simulink model "flightControlSystem"  (R2024b)
settings: Solver=ode3  StartTime=0  StopTime=TFinal  FixedStep=Ts  RelTol=1e-3  EnableMultiTasking=on
undefined symbols (not defined in the file): codertarget, Controller, DiscIntNeverNeededParam, Discrete, Estimator, g, init, K, Sensors, Time, Ts, var_acc_angle_N, var_bias_gyr_N, var_gyro_p_N, Vehicle
libraries: simulink x51, slpidlib x16, sharedtransform x5, ctrlSharedLib x3, eeGeneralControl x1, parrotlib x1
(part 4 of 5)

== system flightControlSystem/Flight Control System/Subsystem/references/Attitude Controller ==
  note: Inner loop PID
      | controls angular velocity
  note: Outer Proportional loop
      | controls the pitch and roll angle
  note: ATTITUDE CONTROL
  refAttitude : Inport
  states_estim : Inport  Port=2
  Angle control loop : slpidlib/PID Controller  Controller=P  Form=Parallel  TimeDomain=Discrete-time  UseExternalTs=off  SampleTime=Ts  IntegratorMethod=Forward Euler  FilterMethod=Forward Euler  ControllerParametersSource=internal  P=2  I=1  UseKiTs=off  D=0  UseExternalDerivativeSource=off  N=100  UseFilter=on  TunerSelectOption=Transfer Function Based (PID Tuner App)  InitialConditionSource=internal  InitialConditionForIntegrator=0  InitialConditionForFilter=0  DifferentiatorICPrevScaledInput=0  ExternalReset=none  TrackingMode=off  Kt=1  LimitOutput=off  SatLimitsSource=internal  UpperSaturationLimit=inf  LowerSaturationLimit=-inf  LinearizeAsGain=on  AntiWindupMode=none  Kb=1  LimitIntegrator=off  UpperIntegratorSaturationLimit=inf  LowerIntegratorSaturationLimit=-inf  PGainOutDataTypeStr=single  PProdOutDataTypeStr=single  POutMin=[]  POutMax=[]  IOutMin=[]  IOutMax=[]  DOutMin=[]  DOutMax=[]  NOutMin=[]  NOutMax=[]  SumOutMin=[]  SumOutMax=[]  SaturationOutMin=[]  SaturationOutMax=[]  PParamMin=[]  PParamMax=[]  IParamMin=[]  IParamMax=[]  DParamMin=[]  DParamMax=[]  NParamMin=[]  NParamMax=[]  KbParamMin=[]  KbParamMax=[]  KtParamMin=[]  KtParamMax=[]  KbOutMin=[]  KbOutMax=[]  KtOutMin=[]  KtOutMax=[]  IntegratorOutMin=[]  IntegratorOutMax=[]  FilterOutMin=[]  FilterOutMax=[]  SumI1OutMin=[]  SumI1OutMax=[]  SumI2OutMin=[]  SumI2OutMax=[]  SumI3OutMin=[]  SumI3OutMax=[]  SumI4OutMin=[]  SumI4OutMax=[]  SumDOutMin=[]  SumDOutMax=[]  DifferentiatorOutMin=[]  DifferentiatorOutMax=[]  FilterDiffOutCoefMin=[]  FilterDiffOutCoefMax=[]  ReciprocalOutMin=[]  ReciprocalOutMax=[]  SumDenOutMin=[]  SumDenOutMax=[]  SumNumOutMin=[]  SumNumOutMax=[]  DivideOutMin=[]  DivideOutMax=[]  UdiffTsProdOutMin=[]  UdiffTsProdOutMax=[]  NTsProdOutMin=[]  NTsProdOutMax=[]  UintegralTsProdOutMin=[]  UintegralTsProdOutMax=[]  UngainTsProdOutMin=[]  UngainTsProdOutMax=[]  ClampingZeroOutDataTypeStr=Inherit: Inherit via back propagation  ClampingZeroOutMin=[]  ClampingZeroOutMax=[]  FilterDenConstantOutDataTypeStr=Inherit: Inherit via back propagation  FilterDenConstantOutMin=[]  FilterDenConstantOutMax=[]  PCopyOutDataTypeStr=Inherit: Inherit via back propagation  PCopyOutMin=[]  PCopyOutMax=[]  NCopyOutDataTypeStr=Inherit: Inherit via back propagation  NCopyOutMin=[]  NCopyOutMax=[]  IntegratorContinuousStateAttributes=''  IntegratorStateMustResolveToSignalObject=off  IntegratorRTWStateStorageClass=Auto  FilterContinuousStateAttributes=''  FilterStateMustResolveToSignalObject=off  FilterRTWStateStorageClass=Auto  ParallelPVariant=InternalParameters  IdealPVariant=Disabled  IVariant=Disabled  DVariant=Disabled  IntegratorVariant=Disabled  SatVariant=Disabled  AWVariant=Disabled  PCopyVariant=Disabled  TRVariant=Disabled  FdbkBlocksVariant=Forward  IdealPFdbkVariant=Disabled  SatFdbkVariant=Disabled  DerivativeFilterVariant=Disabled  NVariant=Disabled  NCopyVariant=Disabled_SignalSpec  FilterICVariant=Disabled  IntegratorICVariant=Disabled  ExternalResetVariant=Disabled  TRSumVariant=Passthrough  SumFdbkVariant=Disabled  SumVariant=Passthrough_P  TsampFilterVariant=InternalTs  TsampNgainVariant=Passthrough  TsampIntegralVariant=Disabled_SignalSpec  ExternalSaturationOutDataTypeStr=Inherit: Same as second input  DerivativeSourceVariant=Disabled  PreIntVariant=InternalPreInt
  Angular velocity control loop : slpidlib/PID Controller  Controller=PID  Form=Parallel  TimeDomain=Discrete-time  UseExternalTs=off  SampleTime=Ts  IntegratorMethod=Forward Euler  FilterMethod=Forward Euler  ControllerParametersSource=internal  P=0.003*[1 0.81]  I=2*0.003*[1 0.81]  UseKiTs=off  D=0.003/25*[1 0.81]  UseExternalDerivativeSource=off  N=70*[1 1]  UseFilter=on  TunerSelectOption=Transfer Function Based (PID Tuner App)  InitialConditionSource=internal  InitialConditionForIntegrator=0  InitialConditionForFilter=0  DifferentiatorICPrevScaledInput=0  ExternalReset=none  TrackingMode=off  Kt=1  LimitOutput=on  SatLimitsSource=internal  UpperSaturationLimit=0.02  LowerSaturationLimit=-0.02  LinearizeAsGain=on  AntiWindupMode=clamping  Kb=1  LimitIntegrator=off  UpperIntegratorSaturationLimit=inf  LowerIntegratorSaturationLimit=-inf  POutMin=[]  POutMax=[]  IOutMin=[]  IOutMax=[]  DOutMin=[]  DOutMax=[]  NOutMin=[]  NOutMax=[]  SumOutMin=[]  SumOutMax=[]  SaturationOutMin=[]  SaturationOutMax=[]  PParamMin=[]  PParamMax=[]  IParamMin=[]  IParamMax=[]  DParamMin=[]  DParamMax=[]  NParamMin=[]  NParamMax=[]  KbParamMin=[]  KbParamMax=[]  KtParamMin=[]  KtParamMax=[]  KbOutMin=[]  KbOutMax=[]  KtOutMin=[]  KtOutMax=[]  IntegratorOutMin=[]  IntegratorOutMax=[]  FilterOutMin=[]  FilterOutMax=[]  SumI1OutMin=[]  SumI1OutMax=[]  SumI2OutMin=[]  SumI2OutMax=[]  SumI3OutMin=[]  SumI3OutMax=[]  SumI4OutMin=[]  SumI4OutMax=[]  SumDOutMin=[]  SumDOutMax=[]  DifferentiatorOutMin=[]  DifferentiatorOutMax=[]  FilterDiffOutCoefMin=[]  FilterDiffOutCoefMax=[]  ReciprocalOutMin=[]  ReciprocalOutMax=[]  SumDenOutMin=[]  SumDenOutMax=[]  SumNumOutMin=[]  SumNumOutMax=[]  DivideOutMin=[]  DivideOutMax=[]  UdiffTsProdOutMin=[]  UdiffTsProdOutMax=[]  NTsProdOutMin=[]  NTsProdOutMax=[]  UintegralTsProdOutMin=[]  UintegralTsProdOutMax=[]  UngainTsProdOutMin=[]  UngainTsProdOutMax=[]  ClampingZeroOutDataTypeStr=Inherit: Inherit via back propagation  ClampingZeroOutMin=[]  ClampingZeroOutMax=[]  FilterDenConstantOutDataTypeStr=Inherit: Inherit via back propagation  FilterDenConstantOutMin=[]  FilterDenConstantOutMax=[]  PCopyOutDataTypeStr=Inherit: Inherit via back propagation  PCopyOutMin=[]  PCopyOutMax=[]  NCopyOutDataTypeStr=Inherit: Inherit via back propagation  NCopyOutMin=[]  NCopyOutMax=[]  IntegratorContinuousStateAttributes=''  IntegratorStateMustResolveToSignalObject=off  IntegratorRTWStateStorageClass=Auto  FilterContinuousStateAttributes=''  FilterStateMustResolveToSignalObject=off  FilterRTWStateStorageClass=Auto  ParallelPVariant=InternalParameters  IdealPVariant=Disabled  IVariant=InternalParameters  DVariant=InternalParameters  IntegratorVariant=Discrete  SatVariant=Enabled  AWVariant=DiscClampingParallel  PCopyVariant=Disabled  TRVariant=Disabled  FdbkBlocksVariant=Forward  IdealPFdbkVariant=Disabled  SatFdbkVariant=Disabled  DerivativeFilterVariant=ForwardEulerFilter  NVariant=InternalParameters  NCopyVariant=Disabled  FilterICVariant=InternalICsFilter  IntegratorICVariant=InternalICs  ExternalResetVariant=Disabled  TRSumVariant=Passthrough  SumFdbkVariant=Disabled  SumVariant=Sum_PID  TsampFilterVariant=InternalTs  TsampNgainVariant=Passthrough  TsampIntegralVariant=Disabled_SignalSpec  ExternalSaturationOutDataTypeStr=Inherit: Same as second input  DerivativeSourceVariant=ErrorSignal  PreIntVariant=InternalPreInt
  Bus Selector1 : BusSelector  OutputSignals=q,p
  Bus Selector3 : BusSelector  OutputSignals=pitch,roll
  Data Type Conversion : DataTypeConversion  SaturateOnIntegerOverflow=off  RndMeth=Floor
  Data Type Conversion1 : DataTypeConversion  SaturateOnIntegerOverflow=off  RndMeth=Floor
  Demux : Demux  Outputs=2
  Demux1 : Demux  Outputs=2
  Mux : Mux  Inputs=2
  Mux1 : Mux  Inputs=2
  Mux2 : Mux  Inputs=2
  Sum1 : Sum  Inputs=|+-
  Sum19 : Sum  Inputs=|+-
  tau_pitch : Outport  VectorParamsAs1DForOutWhenUnconnected=off
  tau_roll : Outport  Port=2  VectorParamsAs1DForOutWhenUnconnected=off
  angular velocity : Outport  Port=3
  wires:
  Sum1/1 -> Angular velocity control loop/1  "pitch/roll error"
  Angle control loop/1 -> Demux/1, Sum1/1
  Sum19/1 -> Angle control loop/1  "pitch/roll error"
  Angular velocity control loop/1 -> Data Type Conversion1/1
  Demux1/2 -> tau_roll/1  "roll acceleration"
  Demux1/1 -> tau_pitch/1  "pitch acceleration"
  Bus Selector3/2 -> Mux/2  "<roll>"
  refAttitude/1 -> Sum19/1
  Bus Selector3/1 -> Mux/1  "<pitch>"
  Bus Selector1/1 -> Mux2/1  "<q>"
  Bus Selector1/2 -> Mux2/2  "<p>"
  Demux/1 -> Mux1/2
  Demux/2 -> Mux1/1
  Mux1/1 -> Data Type Conversion/1
  states_estim/1 -> Bus Selector1/1, Bus Selector3/1
  Mux2/1 -> Sum1/2
  Mux/1 -> Sum19/2
  Data Type Conversion/1 -> angular velocity/1
  Data Type Conversion1/1 -> Demux1/1

== system flightControlSystem/Flight Control System/Subsystem/references/Position Controller ==
  note: Position controller requires good estimate of Yaw orientation to work properly.
      | Incase position control is not needed, the outer loop can be removed and velocity setpoint can be given directly
  note: Inner loop controls linear velocity error
  note: Outer loop controls the position error
  posXY : Inport
  states_estim : Inport  Port=2
  Bus Selector1 : BusSelector  OutputSignals=X,Y
  Bus Selector2 : BusSelector  OutputSignals=dx,dy
  Bus Selector3 : BusSelector  OutputSignals=yaw
  Data Type Conversion : DataTypeConversion  SaturateOnIntegerOverflow=off  RndMeth=Floor
  Data Type Conversion1 : DataTypeConversion  SaturateOnIntegerOverflow=off  RndMeth=Floor
  Gain : Gain  Gain=[-1, 1]
  LPF 8Hz Cutoff Filter to avoid oscillations induced by position controller : DiscreteTransferFcn  Numerator=[1, 1]  Denominator=[1+1/pi/Ts/8, 1-1/pi/Ts/8]
  Mux : Mux  Inputs=2
  Mux1 : Mux  Inputs=2
  Position controller : slpidlib/PID Controller  Controller=P  Form=Parallel  TimeDomain=Discrete-time  UseExternalTs=off  SampleTime=Ts  IntegratorMethod=Forward Euler  FilterMethod=Forward Euler  ControllerParametersSource=internal  P=0.7  I=0.1  UseKiTs=off  D=0  UseExternalDerivativeSource=off  N=100  UseFilter=on  TunerSelectOption=Transfer Function Based (PID Tuner App)  InitialConditionSource=internal  InitialConditionForIntegrator=0  InitialConditionForFilter=0  DifferentiatorICPrevScaledInput=0  ExternalReset=none  TrackingMode=off  Kt=1  LimitOutput=on  SatLimitsSource=internal  UpperSaturationLimit=0.5  LowerSaturationLimit=-0.5  LinearizeAsGain=on  AntiWindupMode=clamping  Kb=1  LimitIntegrator=off  UpperIntegratorSaturationLimit=inf  LowerIntegratorSaturationLimit=-inf  POutMin=[]  POutMax=[]  IOutMin=[]  IOutMax=[]  DOutMin=[]  DOutMax=[]  NOutMin=[]  NOutMax=[]  SumOutMin=[]  SumOutMax=[]  SaturationOutMin=[]  SaturationOutMax=[]  PParamMin=[]  PParamMax=[]  IParamMin=[]  IParamMax=[]  DParamMin=[]  DParamMax=[]  NParamMin=[]  NParamMax=[]  KbParamMin=[]  KbParamMax=[]  KtParamMin=[]  KtParamMax=[]  KbOutMin=[]  KbOutMax=[]  KtOutMin=[]  KtOutMax=[]  IntegratorOutMin=[]  IntegratorOutMax=[]  FilterOutMin=[]  FilterOutMax=[]  SumI1OutMin=[]  SumI1OutMax=[]  SumI2OutMin=[]  SumI2OutMax=[]  SumI3OutMin=[]  SumI3OutMax=[]  SumI4OutMin=[]  SumI4OutMax=[]  SumDOutMin=[]  SumDOutMax=[]  DifferentiatorOutMin=[]  DifferentiatorOutMax=[]  FilterDiffOutCoefMin=[]  FilterDiffOutCoefMax=[]  ReciprocalOutMin=[]  ReciprocalOutMax=[]  SumDenOutMin=[]  SumDenOutMax=[]  SumNumOutMin=[]  SumNumOutMax=[]  DivideOutMin=[]  DivideOutMax=[]  UdiffTsProdOutMin=[]  UdiffTsProdOutMax=[]  NTsProdOutMin=[]  NTsProdOutMax=[]  UintegralTsProdOutMin=[]  UintegralTsProdOutMax=[]  UngainTsProdOutMin=[]  UngainTsProdOutMax=[]  ClampingZeroOutDataTypeStr=Inherit: Inherit via back propagation  ClampingZeroOutMin=[]  ClampingZeroOutMax=[]  FilterDenConstantOutDataTypeStr=Inherit: Inherit via back propagation  FilterDenConstantOutMin=[]  FilterDenConstantOutMax=[]  PCopyOutDataTypeStr=Inherit: Inherit via back propagation  PCopyOutMin=[]  PCopyOutMax=[]  NCopyOutDataTypeStr=Inherit: Inherit via back propagation  NCopyOutMin=[]  NCopyOutMax=[]  IntegratorContinuousStateAttributes=''  IntegratorStateMustResolveToSignalObject=off  IntegratorRTWStateStorageClass=Auto  FilterContinuousStateAttributes=''  FilterStateMustResolveToSignalObject=off  FilterRTWStateStorageClass=Auto  ParallelPVariant=InternalParameters  IdealPVariant=Disabled  IVariant=Disabled  DVariant=Disabled  IntegratorVariant=Disabled  SatVariant=Enabled  AWVariant=Disabled  PCopyVariant=Disabled  TRVariant=Disabled  FdbkBlocksVariant=Forward  IdealPFdbkVariant=Disabled  SatFdbkVariant=Disabled  DerivativeFilterVariant=Disabled  NVariant=Disabled  NCopyVariant=Disabled_SignalSpec  FilterICVariant=Disabled  IntegratorICVariant=Disabled  ExternalResetVariant=Disabled  TRSumVariant=Passthrough  SumFdbkVariant=Disabled  SumVariant=Passthrough_P  TsampFilterVariant=InternalTs  TsampNgainVariant=Passthrough  TsampIntegralVariant=Disabled_SignalSpec  ExternalSaturationOutDataTypeStr=Inherit: Same as second input  DerivativeSourceVariant=Disabled  PreIntVariant=InternalPreInt
  Position error transformation (Earth to Body frame) : MATLAB Function  TreatAsAtomicUnit=on
  Sum1 : Sum  Inputs=|+-
  Sum19 : Sum  Inputs=|+-
  Velocity controller : slpidlib/PID Controller  Controller=PI  Form=Parallel  TimeDomain=Discrete-time  UseExternalTs=off  SampleTime=Ts  IntegratorMethod=Forward Euler  FilterMethod=Forward Euler  ControllerParametersSource=internal  P=0.2  I=0.1  UseKiTs=off  D=0  UseExternalDerivativeSource=off  N=100  UseFilter=on  TunerSelectOption=Transfer Function Based (PID Tuner App)  InitialConditionSource=internal  InitialConditionForIntegrator=0  InitialConditionForFilter=0  DifferentiatorICPrevScaledInput=0  ExternalReset=none  TrackingMode=off  Kt=1  LimitOutput=on  SatLimitsSource=internal  UpperSaturationLimit=20*pi/180  LowerSaturationLimit=-20*pi/180  LinearizeAsGain=on  AntiWindupMode=clamping  Kb=1  LimitIntegrator=off  UpperIntegratorSaturationLimit=inf  LowerIntegratorSaturationLimit=-inf  POutMin=[]  POutMax=[]  IOutMin=[]  IOutMax=[]  DOutMin=[]  DOutMax=[]  NOutMin=[]  NOutMax=[]  SumOutMin=[]  SumOutMax=[]  SaturationOutMin=[]  SaturationOutMax=[]  PParamMin=[]  PParamMax=[]  IParamMin=[]  IParamMax=[]  DParamMin=[]  DParamMax=[]  NParamMin=[]  NParamMax=[]  KbParamMin=[]  KbParamMax=[]  KtParamMin=[]  KtParamMax=[]  KbOutMin=[]  KbOutMax=[]  KtOutMin=[]  KtOutMax=[]  IntegratorOutMin=[]  IntegratorOutMax=[]  FilterOutMin=[]  FilterOutMax=[]  SumI1OutMin=[]  SumI1OutMax=[]  SumI2OutMin=[]  SumI2OutMax=[]  SumI3OutMin=[]  SumI3OutMax=[]  SumI4OutMin=[]  SumI4OutMax=[]  SumDOutMin=[]  SumDOutMax=[]  DifferentiatorOutMin=[]  DifferentiatorOutMax=[]  FilterDiffOutCoefMin=[]  FilterDiffOutCoefMax=[]  ReciprocalOutMin=[]  ReciprocalOutMax=[]  SumDenOutMin=[]  SumDenOutMax=[]  SumNumOutMin=[]  SumNumOutMax=[]  DivideOutMin=[]  DivideOutMax=[]  UdiffTsProdOutMin=[]  UdiffTsProdOutMax=[]  NTsProdOutMin=[]  NTsProdOutMax=[]  UintegralTsProdOutMin=[]  UintegralTsProdOutMax=[]  UngainTsProdOutMin=[]  UngainTsProdOutMax=[]  ClampingZeroOutDataTypeStr=Inherit: Inherit via back propagation  ClampingZeroOutMin=[]  ClampingZeroOutMax=[]  FilterDenConstantOutDataTypeStr=Inherit: Inherit via back propagation  FilterDenConstantOutMin=[]  FilterDenConstantOutMax=[]  PCopyOutDataTypeStr=Inherit: Inherit via back propagation  PCopyOutMin=[]  PCopyOutMax=[]  NCopyOutDataTypeStr=Inherit: Inherit via back propagation  NCopyOutMin=[]  NCopyOutMax=[]  IntegratorContinuousStateAttributes=''  IntegratorStateMustResolveToSignalObject=off  IntegratorRTWStateStorageClass=Auto  FilterContinuousStateAttributes=''  FilterStateMustResolveToSignalObject=off  FilterRTWStateStorageClass=Auto  ParallelPVariant=InternalParameters  IdealPVariant=Disabled  IVariant=InternalParameters  DVariant=Disabled  IntegratorVariant=Discrete  SatVariant=Enabled  AWVariant=DiscClampingParallel  PCopyVariant=Disabled  TRVariant=Disabled  FdbkBlocksVariant=Forward  IdealPFdbkVariant=Disabled  SatFdbkVariant=Disabled  DerivativeFilterVariant=Disabled  NVariant=Disabled  NCopyVariant=Disabled_SignalSpec  FilterICVariant=Disabled  IntegratorICVariant=InternalICs  ExternalResetVariant=Disabled  TRSumVariant=Passthrough  SumFdbkVariant=Disabled  SumVariant=Sum_PI  TsampFilterVariant=InternalTs  TsampNgainVariant=Passthrough  TsampIntegralVariant=Disabled_SignalSpec  ExternalSaturationOutDataTypeStr=Inherit: Same as second input  DerivativeSourceVariant=Disabled  PreIntVariant=InternalPreInt
  Velocity controller1 : slpidlib/PID Controller  Controller=PI  Form=Parallel  TimeDomain=Discrete-time  UseExternalTs=off  SampleTime=Ts  IntegratorMethod=Forward Euler  FilterMethod=Forward Euler  ControllerParametersSource=internal  P=0.7  I=0  UseKiTs=off  D=0  UseExternalDerivativeSource=off  N=100  UseFilter=on  TunerSelectOption=Transfer Function Based (PID Tuner App)  InitialConditionSource=internal  InitialConditionForIntegrator=0  InitialConditionForFilter=0  DifferentiatorICPrevScaledInput=0  ExternalReset=none  TrackingMode=off  Kt=1  LimitOutput=on  SatLimitsSource=internal  UpperSaturationLimit=20*pi/180  LowerSaturationLimit=-20*pi/180  LinearizeAsGain=on  AntiWindupMode=clamping  Kb=1  LimitIntegrator=off  UpperIntegratorSaturationLimit=inf  LowerIntegratorSaturationLimit=-inf  POutMin=[]  POutMax=[]  IOutMin=[]  IOutMax=[]  DOutMin=[]  DOutMax=[]  NOutMin=[]  NOutMax=[]  SumOutMin=[]  SumOutMax=[]  SaturationOutMin=[]  SaturationOutMax=[]  PParamMin=[]  PParamMax=[]  IParamMin=[]  IParamMax=[]  DParamMin=[]  DParamMax=[]  NParamMin=[]  NParamMax=[]  KbParamMin=[]  KbParamMax=[]  KtParamMin=[]  KtParamMax=[]  KbOutMin=[]  KbOutMax=[]  KtOutMin=[]  KtOutMax=[]  IntegratorOutMin=[]  IntegratorOutMax=[]  FilterOutMin=[]  FilterOutMax=[]  SumI1OutMin=[]  SumI1OutMax=[]  SumI2OutMin=[]  SumI2OutMax=[]  SumI3OutMin=[]  SumI3OutMax=[]  SumI4OutMin=[]  SumI4OutMax=[]  SumDOutMin=[]  SumDOutMax=[]  DifferentiatorOutMin=[]  DifferentiatorOutMax=[]  FilterDiffOutCoefMin=[]  FilterDiffOutCoefMax=[]  ReciprocalOutMin=[]  ReciprocalOutMax=[]  SumDenOutMin=[]  SumDenOutMax=[]  SumNumOutMin=[]  SumNumOutMax=[]  DivideOutMin=[]  DivideOutMax=[]  UdiffTsProdOutMin=[]  UdiffTsProdOutMax=[]  NTsProdOutMin=[]  NTsProdOutMax=[]  UintegralTsProdOutMin=[]  UintegralTsProdOutMax=[]  UngainTsProdOutMin=[]  UngainTsProdOutMax=[]  ClampingZeroOutDataTypeStr=Inherit: Inherit via back propagation  ClampingZeroOutMin=[]  ClampingZeroOutMax=[]  FilterDenConstantOutDataTypeStr=Inherit: Inherit via back propagation  FilterDenConstantOutMin=[]  FilterDenConstantOutMax=[]  PCopyOutDataTypeStr=Inherit: Inherit via back propagation  PCopyOutMin=[]  PCopyOutMax=[]  NCopyOutDataTypeStr=Inherit: Inherit via back propagation  NCopyOutMin=[]  NCopyOutMax=[]  IntegratorContinuousStateAttributes=''  IntegratorStateMustResolveToSignalObject=off  IntegratorRTWStateStorageClass=Auto  FilterContinuousStateAttributes=''  FilterStateMustResolveToSignalObject=off  FilterRTWStateStorageClass=Auto  ParallelPVariant=InternalParameters  IdealPVariant=Disabled  IVariant=InternalParameters  DVariant=Disabled  IntegratorVariant=Discrete  SatVariant=Enabled  AWVariant=DiscClampingParallel  PCopyVariant=Disabled  TRVariant=Disabled  FdbkBlocksVariant=Forward  IdealPFdbkVariant=Disabled  SatFdbkVariant=Disabled  DerivativeFilterVariant=Disabled  NVariant=Disabled  NCopyVariant=Disabled_SignalSpec  FilterICVariant=Disabled  IntegratorICVariant=InternalICs  ExternalResetVariant=Disabled  TRSumVariant=Passthrough  SumFdbkVariant=Disabled  SumVariant=Sum_PI  TsampFilterVariant=InternalTs  TsampNgainVariant=Passthrough  TsampIntegralVariant=Disabled_SignalSpec  ExternalSaturationOutDataTypeStr=Inherit: Same as second input  DerivativeSourceVariant=Disabled  PreIntVariant=InternalPreInt
  pitch_roll_cmd : Outport  VectorParamsAs1DForOutWhenUnconnected=off
  velocity_ref : Outport  Port=2
  acceleration_ref : Outport  Port=3
  wires:
  Bus Selector2/1 -> Mux1/1  "<dx>"
  states_estim/1 -> Bus Selector2/1, Bus Selector1/1, Bus Selector3/1
  Bus Selector1/1 -> Mux/1  "<X>"
  Bus Selector1/2 -> Mux/2  "<Y>"
  Bus Selector2/2 -> Mux1/2  "<dy>"
  Mux1/1 -> Sum19/2
  Sum19/1 -> Data Type Conversion1/1, Velocity controller/1
  Velocity controller/1 -> LPF 8Hz Cutoff Filter to avoid oscillations induced by position controller/1
  Gain/1 -> pitch_roll_cmd/1  "Pitch,Roll setpoint"
  LPF 8Hz Cutoff Filter to avoid oscillations induced by position controller/1 -> Gain/1
  Position controller/1 -> Data Type Conversion/1, Sum19/1  "Velocity  setpoint"
  Mux/1 -> Sum1/2
  Sum1/1 -> Position error transformation (Earth to Body frame)/2(xy_err_earth)
  Position error transformation (Earth to Body frame)/1(xy_err_body) -> Position controller/1
  posXY/1 -> Sum1/1  "Position setpoint"
  Bus Selector3/1 -> Position error transformation (Earth to Body frame)/1(yaw)  "<yaw>"
  Velocity controller1/1 -> acceleration_ref/1
  Data Type Conversion/1 -> velocity_ref/1
  Data Type Conversion1/1 -> Velocity controller1/1

== system flightControlSystem/Flight Control System/Controller1/Quaternion-based SMC attitude Controller/Angular velocity handling/Angular velocity ==
  note: Outer Proportional loop
      | controls the pitch and roll angle
  refAttitude1 : Inport
  states_estim1 : Inport  Port=2
  Angle control loop : slpidlib/PID Controller  Controller=P  Form=Parallel  TimeDomain=Discrete-time  UseExternalTs=off  SampleTime=Ts  IntegratorMethod=Forward Euler  FilterMethod=Forward Euler  ControllerParametersSource=internal  P=4  I=0  UseKiTs=off  D=0  UseExternalDerivativeSource=off  N=100  UseFilter=on  TunerSelectOption=Transfer Function Based (PID Tuner App)  InitialConditionSource=internal  InitialConditionForIntegrator=0  InitialConditionForFilter=0  DifferentiatorICPrevScaledInput=0  ExternalReset=none  TrackingMode=off  Kt=1  LimitOutput=off  SatLimitsSource=internal  UpperSaturationLimit=inf  LowerSaturationLimit=-inf  LinearizeAsGain=on  AntiWindupMode=none  Kb=1  LimitIntegrator=off  UpperIntegratorSaturationLimit=inf  LowerIntegratorSaturationLimit=-inf  POutMin=[]  POutMax=[]  IOutMin=[]  IOutMax=[]  DOutMin=[]  DOutMax=[]  NOutMin=[]  NOutMax=[]  SumOutMin=[]  SumOutMax=[]  SaturationOutMin=[]  SaturationOutMax=[]  PParamMin=[]  PParamMax=[]  IParamMin=[]  IParamMax=[]  DParamMin=[]  DParamMax=[]  NParamMin=[]  NParamMax=[]  KbParamMin=[]  KbParamMax=[]  KtParamMin=[]  KtParamMax=[]  KbOutMin=[]  KbOutMax=[]  KtOutMin=[]  KtOutMax=[]  IntegratorOutMin=[]  IntegratorOutMax=[]  FilterOutMin=[]  FilterOutMax=[]  SumI1OutMin=[]  SumI1OutMax=[]  SumI2OutMin=[]  SumI2OutMax=[]  SumI3OutMin=[]  SumI3OutMax=[]  SumI4OutMin=[]  SumI4OutMax=[]  SumDOutMin=[]  SumDOutMax=[]  DifferentiatorOutMin=[]  DifferentiatorOutMax=[]  FilterDiffOutCoefMin=[]  FilterDiffOutCoefMax=[]  ReciprocalOutMin=[]  ReciprocalOutMax=[]  SumDenOutMin=[]  SumDenOutMax=[]  SumNumOutMin=[]  SumNumOutMax=[]  DivideOutMin=[]  DivideOutMax=[]  UdiffTsProdOutMin=[]  UdiffTsProdOutMax=[]  NTsProdOutMin=[]  NTsProdOutMax=[]  UintegralTsProdOutMin=[]  UintegralTsProdOutMax=[]  UngainTsProdOutMin=[]  UngainTsProdOutMax=[]  ClampingZeroOutDataTypeStr=Inherit: Inherit via back propagation  ClampingZeroOutMin=[]  ClampingZeroOutMax=[]  FilterDenConstantOutDataTypeStr=Inherit: Inherit via back propagation  FilterDenConstantOutMin=[]  FilterDenConstantOutMax=[]  PCopyOutDataTypeStr=Inherit: Inherit via back propagation  PCopyOutMin=[]  PCopyOutMax=[]  NCopyOutDataTypeStr=Inherit: Inherit via back propagation  NCopyOutMin=[]  NCopyOutMax=[]  IntegratorContinuousStateAttributes=''  IntegratorStateMustResolveToSignalObject=off  IntegratorRTWStateStorageClass=Auto  FilterContinuousStateAttributes=''  FilterStateMustResolveToSignalObject=off  FilterRTWStateStorageClass=Auto  ParallelPVariant=InternalParameters  IdealPVariant=Disabled  IVariant=Disabled  DVariant=Disabled  IntegratorVariant=Disabled  SatVariant=Disabled  AWVariant=Disabled  PCopyVariant=Disabled  TRVariant=Disabled  FdbkBlocksVariant=Forward  IdealPFdbkVariant=Disabled  SatFdbkVariant=Disabled  DerivativeFilterVariant=Disabled  NVariant=Disabled  NCopyVariant=Disabled_SignalSpec  FilterICVariant=Disabled  IntegratorICVariant=Disabled  ExternalResetVariant=Disabled  TRSumVariant=Passthrough  SumFdbkVariant=Disabled  SumVariant=Passthrough_P  TsampFilterVariant=InternalTs  TsampNgainVariant=Passthrough  TsampIntegralVariant=Disabled_SignalSpec  ExternalSaturationOutDataTypeStr=Inherit: Same as second input  DerivativeSourceVariant=Disabled  PreIntVariant=InternalPreInt
  Bus Selector3 : BusSelector  OutputSignals=pitch,roll
  Constant : Constant  Value=0
  Mux : Mux  Inputs=2
  Mux3 : Mux  Inputs=2
  Sum19 : Sum  Inputs=|+-
  omegaref : Outport
  wires:
  Bus Selector3/2 -> Mux3/2  "<roll>"
  refAttitude1/1 -> Sum19/1
  Bus Selector3/1 -> Mux3/1  "<pitch>"
  Sum19/1 -> Angle control loop/1  "pitch/roll error"
  states_estim1/1 -> Bus Selector3/1
  Mux3/1 -> Sum19/2
  Constant/1 -> Mux/2
  Angle control loop/1 -> Mux/1
  Mux/1 -> omegaref/1

== system flightControlSystem/Flight Control System/Controller1/Quaternion-based SMC attitude Controller/Subsystem/quaternion gen ==
  time : Inport
  tm : Inport  Port=2
  vm : Inport  Port=3
  Add : Sum  Inputs=+-
  Add1 : Sum
  Add2 : Sum  Inputs=+-
  Constant : Constant  Value=2
  Constant1 : Constant
  Constant2 : Constant
  Constant3 : Constant
  Divide : Product  Inputs=*/
  Gain : Gain  Gain=-1
  Gain1 : Gain  Gain=1/2
  Gain2 : Gain  Gain=-1
  Math Function : Math
  Math Function1 : Math  Operator=square
  Mux : Mux
  Product : Product
  Square Root : Sqrt
  Subtract : Sum  Inputs=+-
  qd1 : Constant  Value=0
  qd3 : Constant  Value=0
  q : Outport
  wires:
  Math Function/1 -> Add1/2
  Product/1 -> Math Function/1
  Constant2/1 -> Add2/2
  Add1/1 -> Divide/2
  Divide/1 -> Add2/1
  Constant1/1 -> Add1/1
  Constant3/1 -> Subtract/1
  Subtract/1 -> Square Root/1
  qd3/1 -> Mux/4
  Add2/1 -> Gain2/1
  Gain1/1 -> Add/2
  tm/1 -> Gain1/1
  Constant/1 -> Divide/1
  vm/1 -> Gain/1
  Gain2/1 -> Math Function1/1, Mux/1  "qd0"
  Gain/1 -> Product/2
  Add/1 -> Product/1
  Math Function1/1 -> Subtract/2
  Mux/1 -> q/1
  time/1 -> Add/1
  qd1/1 -> Mux/2
  Square Root/1 -> Mux/3  "qd2"

== system flightControlSystem/Flight Control System/State Estimator/SensorPreprocessing/Temperature Compensation/Triggered Subsystem ==
  In1 : Inport
  Trigger : TriggerPort  TriggerType=either  VariantControl=Variant
  Out1 : Outport
  wires:
  In1/1 -> Out1/1

== system flightControlSystem/Flight Control System/State Estimator/XY Position Estimator/EstimatorVelocity/AccelerationHandling ==
  dxy_estimin : Inport
  sensorIMU_datin : Inport  Port=2
  orient_estimin : Inport  Port=3
  Z_estimin : Inport  Port=4
  Add : Sum  Inputs=-+
  Bus Selector1 : BusSelector  OutputSignals=ddx,ddy,ddz
  Deactivate Acceleration If OF is not used due to low altitude : simulink/Logic and Bit Operations/Compare To Constant  relop=<=  const=Estimator.pos.opticalFlowZMax  OutDataTypeStr=boolean
  Logical Operator : Logic  Operator=OR  AllPortsSameDT=off  OutDataTypeStr=boolean
  Mux6 : Mux  Inputs=3
  Product : Product  Inputs=3
  Product1 : Product  Multiplication=Matrix(*)
  Rotation Angles to Direction Cosine Matrix : sharedtransform/Rotation Angles to Direction Cosine Matrix  rotationOrder=ZYX  aMode=aMode
  SelectPlanarddxy : Selector  InputPortWidth=3  IndexOptions=Index vector (dialog)  Indices=[1 2]  OutputSizes=1
  Selector : Selector  InputPortWidth=2  IndexOptions=Index vector (dialog)  Indices=1  OutputSizes=1
  Selector1 : Selector  InputPortWidth=2  IndexOptions=Index vector (dialog)  Indices=2  OutputSizes=1
  do not use acc if optical flow never available (Note OF@60Hz but ZOH to 200!) : simulink/Logic and Bit Operations/Compare To Constant  relop=~=  const=0  OutDataTypeStr=boolean
  do not use acc if optical flow never available (Note OF@60Hz but ZOH to 200!)1 : simulink/Logic and Bit Operations/Compare To Constant  relop=~=  const=0  OutDataTypeStr=boolean
  gainaccinput1 : Gain  OutDataTypeStr=single
  gravity : Constant  Value=[0 0 -g]
  acceleration_world : Outport  OutDataTypeStr=single  VectorParamsAs1DForOutWhenUnconnected=off
  wires:
  do not use acc if optical flow never available (Note OF@60Hz but ZOH to 200!)1/1 -> Logical Operator/2
  do not use acc if optical flow never available (Note OF@60Hz but ZOH to 200!)/1 -> Logical Operator/1
  Logical Operator/1 -> Product/1
  Selector1/1 -> do not use acc if optical flow never available (Note OF@60Hz but ZOH to 200!)1/1
  Selector/1 -> do not use acc if optical flow never available (Note OF@60Hz but ZOH to 200!)/1
  dxy_estimin/1 -> Selector1/1, Selector/1
  Product/1 -> acceleration_world/1
  Deactivate Acceleration If OF is not used due to low altitude/1 -> Product/3
  Z_estimin/1 -> Deactivate Acceleration If OF is not used due to low altitude/1
  Add/1 -> SelectPlanarddxy/1
  Product1/1 -> Add/1
  gravity/1 -> Product1/2
  SelectPlanarddxy/1 -> gainaccinput1/1
  Bus Selector1/3 -> Mux6/3  "<ddz>"
  Bus Selector1/1 -> Mux6/1  "<ddx>"
  sensorIMU_datin/1 -> Bus Selector1/1
  Mux6/1 -> Add/2
  Bus Selector1/2 -> Mux6/2  "<ddy>"
  orient_estimin/1 -> Rotation Angles to Direction Cosine Matrix/1
  Rotation Angles to Direction Cosine Matrix/1 -> Product1/1
  gainaccinput1/1 -> Product/2

== system flightControlSystem/Flight Control System/State Estimator/XY Position Estimator/EstimatorVelocity/Angular velocity compensation for optical flow ==
  note: Optical flow readings are affected by both linear and angular velocity of the drone. We need to subtract the effect of angular velocity before using the flow data
  z_estimate : Inport
  Angular velocity w/o bias : Inport  Port=2
  Abs : Abs  SaturateOnIntegerOverflow=off
  Data Type Conversion : DataTypeConversion  SaturateOnIntegerOverflow=off  RndMeth=Floor
  Demux : Demux  Outputs=2
  Gain1 : Gain  Gain=-1
  Mux : Mux  Inputs=2
  Selector : Selector  InputPortWidth=3  IndexOptions=Index vector (dialog)  Indices=[1 2]  OutputSizes=1
  prod : Product  Inputs=**
  angular velocity correction : Outport
  wires:
  Gain1/1 -> Mux/1
  Mux/1 -> Data Type Conversion/1
  Demux/2 -> Gain1/1
  Data Type Conversion/1 -> angular velocity correction/1
  prod/1 -> Demux/1
  z_estimate/1 -> Abs/1
  Demux/1 -> Mux/2
  Selector/1 -> prod/2
  Abs/1 -> prod/1
  Angular velocity w/o bias/1 -> Selector/1

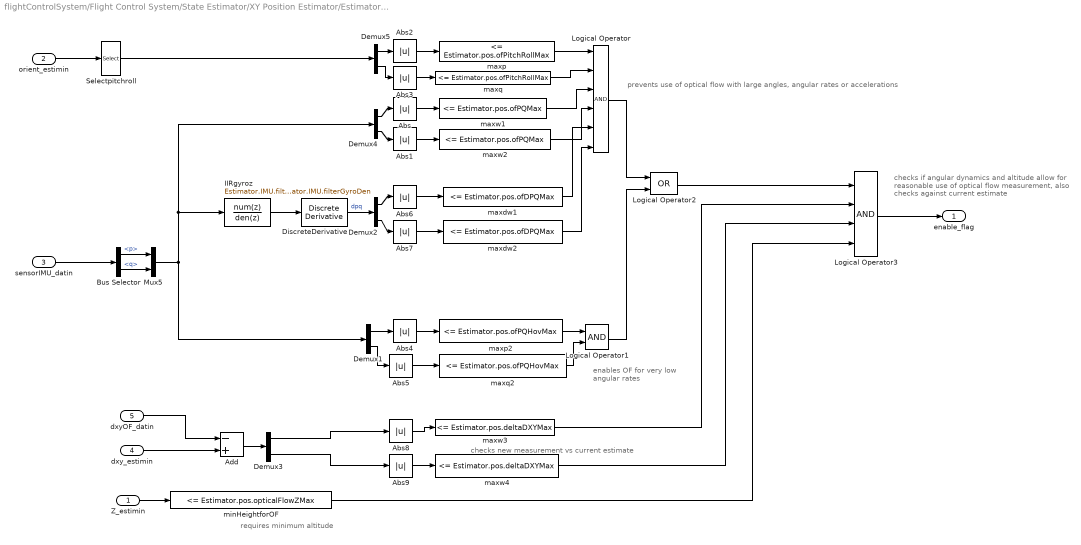
== system flightControlSystem/Flight Control System/State Estimator/XY Position Estimator/EstimatorVelocity/DataHandling ==
  note: prevents use of optical flow with large angles, angular rates or accelerations
  note: enables OF for very
      | low angular rates
  note: checks if angular dynamics and altitude allow for
      | reasonable use of optical flow measurement,
      | also checks against current estimate
  note: checks new measurement vs current estimate
  note: requires minimum altitude
  Z_estimin : Inport
  orient_estimin : Inport  Port=2
  sensorIMU_datin : Inport  Port=3
  dxy_estimin : Inport  Port=4
  dxyOF_datin : Inport  Port=5
  Abs{,1..9} (10 alike) : Abs  SaturateOnIntegerOverflow=off
  Add : Sum  Inputs=-+
  Bus Selector : BusSelector  OutputSignals=p,q
  Demux{1..5} (5 alike) : Demux  Outputs=2
  DiscreteDerivative : simulink/Discrete/Discrete Derivative  gainval=1.0  ICPrevScaledInput=0.0  OutMin=[]  OutMax=[]  OutDataType=fixdt(1, 16)  OutScaling=2^-10  DoSatur=off
  IIRgyroz : DiscreteFilter  Numerator=Estimator.IMU.filterGyroNum  Denominator=Estimator.IMU.filterGyroDen
  Logical Operator : Logic  Inputs=6  AllPortsSameDT=off  OutDataTypeStr=boolean
  Logical Operator1 : Logic  AllPortsSameDT=off  OutDataTypeStr=boolean
  Logical Operator2 : Logic  Operator=OR  AllPortsSameDT=off  OutDataTypeStr=boolean
  Logical Operator3 : Logic  Inputs=4  AllPortsSameDT=off  OutDataTypeStr=boolean
  Mux5 : Mux  Inputs=2
  Selectpitchroll : Selector  InputPortWidth=3  IndexOptions=Index vector (dialog)  Indices=[2 3]  OutputSizes=1
  maxdw1 : simulink/Logic and Bit Operations/Compare To Constant  relop=<=  const=Estimator.pos.ofDPQMax  OutDataTypeStr=boolean
  maxdw2 : simulink/Logic and Bit Operations/Compare To Constant  relop=<=  const=Estimator.pos.ofDPQMax  OutDataTypeStr=boolean
  maxp : simulink/Logic and Bit Operations/Compare To Constant  relop=<=  const=Estimator.pos.ofPitchRollMax  OutDataTypeStr=boolean
  maxp2 : simulink/Logic and Bit Operations/Compare To Constant  relop=<=  const=Estimator.pos.ofPQHovMax  OutDataTypeStr=boolean
  maxq : simulink/Logic and Bit Operations/Compare To Constant  relop=<=  const=Estimator.pos.ofPitchRollMax  OutDataTypeStr=boolean
  maxq2 : simulink/Logic and Bit Operations/Compare To Constant  relop=<=  const=Estimator.pos.ofPQHovMax  OutDataTypeStr=boolean
  maxw1 : simulink/Logic and Bit Operations/Compare To Constant  relop=<=  const=Estimator.pos.ofPQMax  OutDataTypeStr=boolean
  maxw2 : simulink/Logic and Bit Operations/Compare To Constant  relop=<=  const=Estimator.pos.ofPQMax  OutDataTypeStr=boolean
  maxw3 : simulink/Logic and Bit Operations/Compare To Constant  relop=<=  const=Estimator.pos.deltaDXYMax  OutDataTypeStr=boolean
  maxw4 : simulink/Logic and Bit Operations/Compare To Constant  relop=<=  const=Estimator.pos.deltaDXYMax  OutDataTypeStr=boolean
  minHeightforOF : simulink/Logic and Bit Operations/Compare To Constant  relop=<=  const=Estimator.pos.opticalFlowZMax  OutDataTypeStr=boolean
  enable_flag : Outport  VectorParamsAs1DForOutWhenUnconnected=off
  wires:
  minHeightforOF/1 -> Logical Operator3/4
  IIRgyroz/1 -> DiscreteDerivative/1
  Mux5/1 -> Demux1/1, Demux4/1, IIRgyroz/1
  maxw4/1 -> Logical Operator3/3
  maxw3/1 -> Logical Operator3/2
  dxyOF_datin/1 -> Add/1
  Demux3/2 -> Abs9/1
  Demux3/1 -> Abs8/1
  dxy_estimin/1 -> Add/2
  Add/1 -> Demux3/1
  Abs9/1 -> maxw4/1
  Abs8/1 -> maxw3/1
  Logical Operator2/1 -> Logical Operator3/1
  Logical Operator3/1 -> enable_flag/1
  DiscreteDerivative/1 -> Demux2/1  "dpq"
  Demux2/2 -> Abs7/1
  Demux2/1 -> Abs6/1
  Abs7/1 -> maxdw2/1
  Abs6/1 -> maxdw1/1
  Logical Operator1/1 -> Logical Operator2/2
  Demux1/2 -> Abs5/1
  Demux1/1 -> Abs4/1
  Abs5/1 -> maxq2/1
  Abs4/1 -> maxp2/1
  Abs3/1 -> maxq/1
  Abs2/1 -> maxp/1
  Demux4/2 -> Abs1/1
  Demux4/1 -> Abs/1
  Abs1/1 -> maxw2/1
  Abs/1 -> maxw1/1
  Z_estimin/1 -> minHeightforOF/1
  Logical Operator/1 -> Logical Operator2/1
  maxw1/1 -> Logical Operator/3
  Bus Selector/1 -> Mux5/1  "<p>"
  Selectpitchroll/1 -> Demux5/1
  sensorIMU_datin/1 -> Bus Selector/1
  maxq2/1 -> Logical Operator1/2
  Bus Selector/2 -> Mux5/2  "<q>"
  maxp/1 -> Logical Operator/1
  maxw2/1 -> Logical Operator/4
  orient_estimin/1 -> Selectpitchroll/1
  maxdw1/1 -> Logical Operator/5
  maxdw2/1 -> Logical Operator/6
  maxq/1 -> Logical Operator/2
  Demux5/1 -> Abs2/1
  Demux5/2 -> Abs3/1
  maxp2/1 -> Logical Operator1/1

== system flightControlSystem/Flight Control System/State Estimator/XY Position Estimator/EstimatorVelocity/XY velocity w//o angular velocity compensation ==
  note: Optical flow raw readings are converted to velocity in m/s based on the estimated altitude
  optical_flow : Inport
  z_estimate : Inport  Port=2
  " " : Product  Inputs=**
  Compare To Constant : simulink/Logic and Bit Operations/Compare To Constant  relop=<  const=200*4  OutDataTypeStr=boolean
  Counter Free-Running : simulink/Sources/Counter Free-Running  NumBits=32  tsamp=-1
  Gain : Gain  Gain=-1
  Select dxy : Selector  InputPortWidth=3  IndexOptions=Index vector (dialog)  Indices=[1 2]  OutputSizes=1
  Switch : Switch  Criteria=u2 > Threshold  SaturateOnIntegerOverflow=off  InputSameDT=off
  opticalFlowErrorCorrect : Gain  Gain=1.15
  optical_flow_dx_dy : Outport
  wires:
  Select dxy/1 -> optical_flow_dx_dy/1  "optical_flow_dx_dy"
  " "/1 -> opticalFlowErrorCorrect/1
  opticalFlowErrorCorrect/1 -> Switch/3
  Gain/1 -> " "/2
  Switch/1 -> Select dxy/1
  Counter Free-Running/1 -> Compare To Constant/1
  Compare To Constant/1 -> Switch/2
  optical_flow/1 -> " "/1, Switch/1
  z_estimate/1 -> Gain/1

== matlab function flightControlSystem/Flight Control System/State Estimator/Attitude EKF quaternion + yaw using basic estimator /MATLAB Function ==
  data: q output; P output; q_prec input; P_prec input; acc input; gyro input; yaw output; pitch output; roll output; should_reset input
function [q, P, yaw ,pitch, roll] = fnc(q_prec, P_prec, acc, gyro, should_reset)


if should_reset
    P_prec = eye(4);
    q_prec = [1,0,0,0]';
end

wx = gyro(1);
wy = gyro(2);
wz = gyro(3);

dt= 0.0025;

noise_gyro = 0.3 ;
noise_acc = 0.5 ;

w= [wx;wy;wz];

qw_p=q_prec(1);
qx_p=q_prec(2);
qy_p=q_prec(3);
qz_p=q_prec(4);

Omega = [0,-wx,-wy,-wz;
    wx,0,wz,-wy;
    wy,-wz,0,wx;
    wz,wy,-wx,0];

if norm(w)==0 
    q=q_prec;
    P=P_prec;
    w = q(1);
    x = q(2);
    y = q(3);
    z = q(4);
    yaw = atan2(2 * (w * z + x * y), 1 - 2 * (y^2 + z^2));
    pitch = asin(2 * (w * y - x * z));
    roll = atan2(2 * (w * x + y * z), 1 - 2 * (x^2 + y^2));


else 
    % 2 option pour q_hat 
    qhat = ( cos(norm(w)*dt/2)*eye(4) + 2/norm(w)*sin(norm(w)*dt/2)*Omega)* q_prec ;

    % qhat = (eye(4) + dt/2*Omega)*q_prec ; 

    qhatw = qhat(1);
    qhatx = qhat(2);
    qhaty = qhat(3);
    qhatz = qhat(4);

    F=dt/2*[2/dt,-wx,-wy,-wz;
        wx,2/dt,wz,-wy;
        wy,-wz,2/dt,wx;
        wz,wy,-wx,2/dt];

    Wt = dt/2*[-qx_p,-qy_p,-qz_p;
        qw_p,-qz_p,qy_p;
        qz_p,qw_p,-qx_p;
        -qy_p,qx_p,qw_p];
    Qt = (noise_gyro^2)* (Wt)*(Wt');

    P_hat = F*P_prec*F'+Qt;

    z = [acc(1),acc(2),acc(3)]';
    z = z/norm(z);

    g=-1; %ned ou enu ?

    h= 2*[g*(qhatx*qhatz-qhatw*qhaty);
       g*(qhatw*qhatx+qhaty*qhatz);
       g*(.5-qhatx^2-qhaty^2)];

    h = h/norm(h);

    H = 2* [-g*qhaty, g*qhatz, -g*qhatw, g*qhatx;
       g*qhatx, g*qhatw,g*qhatz, g*qhaty;
       g*qhatw, -g*qhatx, -g*qhaty, g*qhatz];

    R = noise_acc^2 * eye(3);

    v = z - h ;
    S= H*P_hat*H' + R ;
    invS = inv(S);
    K=P_hat*H'*invS;
    q = qhat + K*v ;

    P = (eye(4)-K*H)*P_hat;

    q= q/norm(q);

    w = q(1);
    x = q(2);
    y = q(3);
    z = q(4);

    % Compute Yaw (ψ) - Rotation around Z-axis
    yaw = atan2(2 * (w * z + x * y), 1 - 2 * (y^2 + z^2));

    % Compute Pitch (θ) - Rotation around Y-axis
    pitch = asin(2 * (w * y - x * z));  % Beware of gimbal lock if |pitch| = 90°

    % Compute Roll (φ) - Rotation around X-axis
    roll = atan2(2 * (w * x + y * z), 1 - 2 * (x^2 + y^2));
end

== matlab function flightControlSystem/Flight Control System/Controller1/Position SMC/MATLAB Function ==
  data: pos_ref input; pitch output; pos input; vel input; yaw input; C input; m input; U1 input; K input; roll output; s output; phi input
function [pitch,roll, s] = pos_SMC(pos_ref, pos, vel, yaw, C,m,U1,K, phi)
e= pos_ref - pos ; 
edot = - vel ;
s = edot + C*e;
xdotdot=0 ;
if abs(s(1)) > phi(1)
    sat_s1 = tanh(s(1));
else
    sat_s1 = s(1) / phi(1);
end

if abs(s(2)) > phi(2)
    sat_s2 = tanh(s(2));
else
    sat_s2 = s(2) / phi(2);
end

% Compute control inputs
Ux = (m / U1) * (K(1,1)*sat_s1 + K(1,2)*s(1) + xdotdot + C(1,1)*edot(1));
Uy = (m / U1) * (K(2,2)*sat_s2 + K(2,1)*s(2) + xdotdot + C(2,2)*edot(2));

% Compute roll and pitch
roll = asin(min(max(Ux*sin(yaw) - Uy*cos(yaw), -1), 1));
pitch = asin(min(max((Ux*cos(yaw) + Uy*sin(yaw)) / cos(roll), -1), 1));

== matlab function flightControlSystem/Flight Control System/Controller1/Position LQR/Position error transformation (Earth to Body frame) ==
  data: yaw input; xy_err_earth input; xy_err_body output
function xy_err_body = fcn(yaw,xy_err_earth)

transformation = [cos(yaw), sin(yaw); -sin(yaw),  cos(yaw)];
xy_err_body = transformation * xy_err_earth;


end

== matlab function flightControlSystem/Flight Control System/Controller1/Quaternion Pos SMC/Quaternion-based positon control ==
  data: pos_ref input; pos input; vel input; acc input; lambda input; Ks input; ki output; ki_dot output; f output; q input; m input
function [ki, ki_dot, f] = Quat_POS_SMC(pos_ref, pos, vel, acc, lambda, Ks, q, m)

g = 9.81;

% Error terms
pos_error = pos - pos_ref;
v_error = vel;
a_error = acc;
% Sliding surface
s = v_error + lambda * pos_error;
s_dot = Ks * tanh(s/2);
% Normalize quaternion
q = q / norm(q);

% Control input
ki = single(m * (-lambda * v_error + g * [0; 0; 1] - s_dot))


sech_sq = (1 ./ cosh(s)).^2;

ki_dot = m * ( -Ks * (sech_sq .* s_dot));

% Quaternion rotation of body Z-axis [0; 0; 1] into NED frame (right-hand rule)
quat_f = single([0; 0; 0]);
quat_f(1) = 2 * (q(2) * q(4) - q(1) * q(3));                         % x
quat_f(2) = 2 * (q(1) * q(2) + q(3) * q(4));                         % y
quat_f(3) = q(1)^2 - q(2)^2 - q(3)^2 + q(4)^2;                       % z

% Total thrust (scalar)
f = dot(ki, quat_f);

== matlab function flightControlSystem/Flight Control System/Controller1/Quaternion Pos SMC/Quaternion trajectory generation ==
  data: k input; qd output; k_dot input; b1r input; omega_d output
function [qd, omega_d] = computeAttitudeTrajectory_NED(k, k_dot, b1r)
% Normalize k to get b3d (now downward in NED)
b3d = k / norm(k);

% v = cross(b3d, b1d) [NED: b1d = North, b3d = Down → b2d = East]
v = cross(b3d, b1r);
v_norm = norm(v);
b2d = v / v_norm;

% b1d_prime = cross(b2d, b3d) [Ensures orthonormal NED triad]
b1d_prime = cross(b2d, b3d);

% Build desired rotation matrix Rd (NED frame)
Rd = [b1d_prime, -b2d, -b3d]

% --- Derivatives remain mathematically identical but now in NED ---
k_norm = norm(k);
k_dot_proj = dot(k, k_dot);
k_dot_norm_sq = k_dot_proj / (k_norm^3);
b3d_dot = (k_dot / k_norm - k_dot_norm_sq * k);
v_dot = cross(b3d_dot, b1r);
v_cross_vdot = dot(v, v_dot);
b2d_dot = (v_dot / v_norm) - ((v_cross_vdot / v_norm^3) * v);
b1d_dot = cross(b2d_dot, b3d) + cross(b2d, b3d_dot);

% Rd_dot in NED
Rd_dot = [b1d_dot, b2d_dot, b3d_dot];

% Extract angular velocity (NED convention)
omega_d_hat = Rd' * Rd_dot;
omega_d = [omega_d_hat(3,2); omega_d_hat(1,3); omega_d_hat(2,1)];

% Convert Rd to quaternion (scalar-first, MATLAB convention)
qd = rotm2quat(Rd)
end

== matlab function flightControlSystem/Flight Control System/State Estimator/Altitude Estimator1/MATLAB Function ==
  data: z_meas input; u input; x_est output; Q input; R input; x0 input; P0 input; Enable input
function x_est = CustomEKF(z_meas, u, Q, R, x0, P0, Enable)
% Inputs:
% z_meas : scalar measurement (altitude)
% u      : scalar acceleration input (ddz)
% Q, R   : covariance matrices
% x0     : initial state [z; dz; bias]
% P0     : initial covariance matrix
% Enable : logical (1 = run, 0 = hold)

persistent x P
Ts = 0.005;

if isempty(x)
    x = x0;
end
if isempty(P)
    P = P0;
end

if 1
    %% === Prediction Step ===
    % State unpack
    z = x(1);
    dz = x(2);

    % Input
    ddz = u;

    % Predict state using nonlinear model
    z_pred  = z + dz * Ts;
    dz_pred = dz + (ddz) * Ts;

    x_pred = [z_pred; dz_pred];

    % Jacobian of state transition (F)
    F = [1, Ts;
         0,  1];

    % Predict covariance
    P_pred = F * P * F' + Q;

    %% === Update Step ===
    % Measurement model: y = x(1)
    H = [1, 0];

    % Measurement residual
    y_pred = x_pred(1);
    y = z_meas;
    innovation = y - y_pred;

    % Kalman Gain
    S = H * P_pred * H' + R;
    K = P_pred * H' / S;

    % Update state
    x = x_pred + K * innovation;

    % Update covariance
    P = (eye(2) - K * H) * P_pred;
end

% Output state and covariance
x_est = x;

== matlab function flightControlSystem/Flight Control System/Controller1/Quaternion-based SMC attitude Controller/Subsystem/MATLAB Function1 ==
  data: q input; t input; omega output; tm input; vm input; dq output
function [omega, dq] = quat_to_omega(q, t, tm, vm)
    dq = [0; 0; 0; 0];
    dq(1) = -(2 * vm * exp(-vm * (t - tm / 2))) / (exp(-vm * (t - tm / 2)) + 1)^2;
    dq(2) = 0;
    dq(3) = (-q(1) / sqrt(1 - q(1)^2)) * dq(1);
    q_conj = [q(1); -q(2:4)];
    
    % Quaternion multiplication: dq ⊗ q_conj
    dq_qinv = quatmultiply(dq', q_conj');
    
    % Angular velocity (vector part of result times 2)
    omega = 2 * dq_qinv(2:4)';
end

== matlab function flightControlSystem/Flight Control System/Subsystem/Sliding mode controller ==
  data: x input; x_dot input; ref input; ref_dot input; ref_dot_dot input; U output; m input; I input; L input; Jr input; omega input; Err output; rho1 input; Int input
function [U, Err] = Sliding_Mode_Controller(x, x_dot, ref, ref_dot, ref_dot_dot, m, I, L, Jr, omega, rho1, Int)
    
    % x = [x y z phi theta psi]
    r = 0.01;
    g = 9.81;
    Ix = I(1,1);
    Iy = I(2,2);
    Iz = I(3,3);
    K = [0, 0, 0, 0, 0, 0;...
        0, 0, 0, 0, 0, 0;...
        0, 0, 3.5, 0, 0, 0;...
        0, 0, 0, 20, 0, 0;
        0, 0, 0, 0, 0, 0;...
        0, 0, 0, 0, 0 ,0;
        ];
    C = [0, 0, 0, 0, 0, 0;...
        0, 0, 0, 0, 0, 0;...
        0, 0, 2.5, 0, 0, 0;...
        0, 0, 0, 2.5, 0, 0;
        0, 0, 0, 0, 0, 0;...
        0, 0, 0, 0, 0 ,0;
        ];
    phi = x(4);
    theta = x(5);
    psi = x(6);

    psi_ref = ref(6);

    f1 = r/m;
    f2 = r/m;
    f3 = r/m + g;
    f4 = x_dot(5) * x_dot(6) * ((Iy - Iz)/Ix) - (Jr/Ix)*omega*x_dot(5);
    f5 = x_dot(4) * x_dot(6) * ((Iz - Ix)/Iy) + (Jr/Iy)*omega*x_dot(4);
    f6 = x_dot(4) * x_dot(5) * ((Ix - Iy)/Iz);

    g1 = -(cos(phi) * sin(theta) * cos(psi) + sin(phi) * sin(psi)) / m;
    g2 = -(cos(phi) * sin(theta) * sin(psi) - sin(phi) * cos(psi)) / m;
    g3 = (cos(phi) * cos(theta)) / m;
    g4 = L/Ix;
    g5 = L/Iy;
    g6 = 1/Iz;
    
    
    G = [g1, 0, 0, 0;...
        g2, 0, 0, 0;...
        g3, 0, 0, 0;...
        0, g4, 0, 0;...
        0, 0, g5, 0;...
        0, 0, 0, g6;
        ];
    F = [f1, f2, f3, f4, f5, f6]';
    
    % if (omega ~= 0)
    %     U1 = rho1*(omega);
    %     ref(4) = (m/U1) * (ref_dot_dot(1) * sin(psi_ref) - ref_dot_dot(2) * cos(psi_ref));
    %     ref(5) = (m/U1) * (ref_dot_dot(1) * cos(psi_ref) + ref_dot_dot(2) * sin(psi_ref));
    % end
    
    E = (x-ref);
    Err = E;

    T = [cos(psi_ref), sin(psi_ref); -sin(psi_ref),  cos(psi_ref)];
    E(1:2) = T*E(1:2);
    
    E_dot = x_dot - ref_dot;
    S = C*(E) + E_dot
    
    if (abs(S(3)) < 1.5)
        K(3,3) = 3;
    else
        K(3,3) = K(3,3);
    end
    

    

    Url = -pinv(G) * K * tanh(S)
    Ueq = +pinv(G) * (C*E_dot + F - ref_dot_dot)
    U = (Ueq + Url);
end

== matlab function flightControlSystem/Flight Control System/Controller/Position Controller/Position error transformation (Earth to Body frame) ==
  data: yaw input; xy_err_earth input; xy_err_body output
function xy_err_body = fcn(yaw,xy_err_earth)

transformation = [cos(yaw), sin(yaw); -sin(yaw),  cos(yaw)];
xy_err_body = transformation * xy_err_earth;


end

== matlab function flightControlSystem/Flight Control System/Subsystem/ControlInputToOmega ==
  data: U input; omega output; rho1 input; rho2 input; L input
function omega = ControlInputToOmega(U, rho1, rho2, L)

    A = [rho1, rho1, rho1, rho1;
        rho1, -rho1, -rho1, rho1;
        rho1, rho1, -rho1, -rho1;
        -rho2, rho2, -rho2, rho2];
    b = U;
    omega_sq = A\b;

    omega_sq(find(omega_sq < 0)) = 0;
    omega = sqrt(omega_sq);
end

== matlab function flightControlSystem/Flight Control System/Subsystem/references/Position Controller/Position error transformation (Earth to Body frame) ==
  data: yaw input; xy_err_earth input; xy_err_body output
function xy_err_body = fcn(yaw,xy_err_earth)

transformation = [cos(yaw), sin(yaw); -sin(yaw),  cos(yaw)];
xy_err_body = transformation * xy_err_earth;


end

== matlab function flightControlSystem/Flight Control System/Controller1/Position Controller/Position error transformation (Earth to Body frame) ==
  data: yaw input; xy_err_earth input; xy_err_body output
function xy_err_body = fcn(yaw,xy_err_earth)

transformation = [cos(yaw), sin(yaw); -sin(yaw),  cos(yaw)];
xy_err_body = transformation * xy_err_earth;


end

== matlab function flightControlSystem/Flight Control System/Controller1/Quaternion-based SMC attitude Controller/MATLAB Function ==
  data: q_d input; tau output; q input; omega_d input; omega input; J input; Lambda input; K input; Ks input
function tau = quaternion_smc(q_d, q, omega_d, omega, J, Lambda, K, Ks)
    % Quaternion-Based Sliding Mode Control (SMC) for Quadrotor
    % Inputs:
    %   q_d - Desired quaternion [q0, q1, q2, q3]
    %   q   - Current quaternion [q0, q1, q2, q3]
    %   omega_d - Desired angular velocity [ωx, ωy, ωz] (rad/s)
    %   omega - Current angular velocity [ωx, ωy, ωz] (rad/s)
    %   J - Inertia matrix [3x3]
    %   Lambda - Sliding gain matrix [3x3]
    %   K - Control gain matrix [3x3]
    %   Ks - Discontinuous control gain matrix [3x3]
    % Output:
    %   tau - Control torques [τx, τy, τz] (Nm)

    % Ensure quaternions are normalized
    q_d = q_d / norm(q_d);
    q = q / norm(q);


    % Compute Quaternion Error: q_e = q_d^(-1) ⊗ q
    q_d_inv = [q_d(1), -q_d(2), -q_d(3), -q_d(4)]; % Quaternion inverse
    q_e = quatmultiply(q_d_inv, q); % Quaternion error (MATLAB built-in)
    
    % Extract vector part of quaternion error
    q_ev = q_e(2:4); % [q_e1, q_e2, q_e3] (3x1 vector)
    
    
    % Compute Sliding Surface: S = (ω - ω_d) + Λ * q_ev
    S = (omega - omega_d) + Lambda * sign(q(1))* q_ev';

    % Compute Control Torque: τ = J * (-K * S - Ks * sign(S)) - ω × (Jω)
    tau = -K * S - Ks * tanh(S./4);
    tau = J * tau - cross(omega, J * omega);

end
